simulink model "POLAR_2RP_IK"  (R2019b)
settings: Solver=VariableStepAuto  StartTime=0.0  StopTime=6.0  RelTol=1e-3
undefined symbols (not defined in the file): q_0_polar_2RP, timeStep
settings Model: Creator=simone  LastModifiedBy=simone

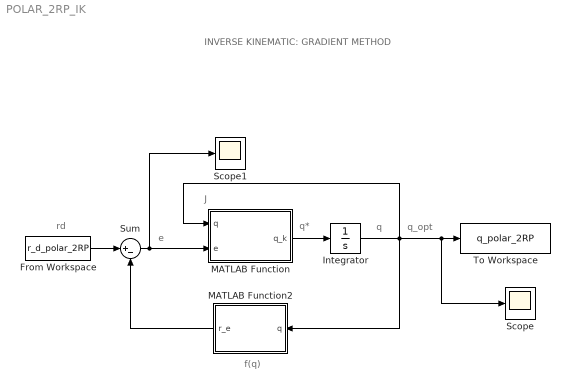
== system POLAR_2RP_IK ==
  note: INVERSE KINEMATIC: GRADIENT METHOD
  note: e
  note: q_opt
  note: q
  note: q*
  note: f(q)
  note: J
  note: rd
  From Workspace : FromWorkspace  VariableName=r_d_polar_2RP  SampleTime=timeStep
  Integrator : Integrator  InitialCondition=q_0_polar_2RP
  MATLAB Function : MATLAB Function  TreatAsAtomicUnit=on
  MATLAB Function2 : MATLAB Function  TreatAsAtomicUnit=on
  Scope : Scope
  Scope1 : Scope
  Sum : Sum  Inputs=|+-
  To Workspace : ToWorkspace  VariableName=q_polar_2RP  SaveFormat=Timeseries  SampleTime=-1
  wires:
  From Workspace/1 -> Sum/1
  MATLAB Function/1(q_k) -> Integrator/1
  Integrator/1 -> MATLAB Function/1(q), MATLAB Function2/1(q), To Workspace/1, Scope/1
  MATLAB Function2/1(r_e) -> Sum/2
  Sum/1 -> Scope1/1, MATLAB Function/2(e)

== matlab function POLAR_2RP_IK/MATLAB Function ==
  data: q_k output; q input; e input
function q_k = J_r(q,e)
% GRADIENT
alpha =  0.7;
J_q = [-q(3)*sin(q(1))*sin(q(2)) q(3)*cos(q(1))*cos(q(2)) cos(q(1))*sin(q(2));
    q(3)*cos(q(1))*sin(q(2)) q(3)*cos(q(2))*sin(q(1)) sin(q(1))*sin(q(2));
    0 -q(3)*sin(q(2)) cos(q(2))];
q_k = alpha * J_q' * e;

% NEWTON
% Jq = [-q(3)*sin(q(1))*sin(q(2)) q(3)*cos(q(1))*cos(q(2)) cos(q(1))*sin(q(2));
%     q(3)*cos(q(1))*sin(q(2)) q(3)*cos(q(2))*sin(q(1)) sin(q(1))*sin(q(2));
%     0 -q(3)*sin(q(2)) cos(q(2))];
% q_k =  inv(Jq) * e;

== matlab function POLAR_2RP_IK/MATLAB Function2 ==
  data: r_e output; q input
function r_e = F_r(q)
%POLAR ROBOT (2R P)
r_e = [q(3)*cos(q(1))*sin(q(2));
    q(3)*sin(q(1))*sin(q(2));
    q(3)*cos(q(2))+0.5];
